simulink model "Test_Bit_Demultiplexer_1_to_4"  (Simulink 8.1)
settings: Solver=ode45  StartTime=0.0  StopTime=len  RelTol=1e-3
libraries: commutil2 x3, Bit_Demultiplexers_Lib x1
settings Model: Creator=N  LastModifiedBy=uzivatel
settings DataIOCC: LimitDataPoints=off  SignalLoggingSaveFormat=Dataset
settings OptimizationCC: ExpressionDepthLimit=128
settings DebuggingCC: UnderspecifiedInitializationDetection=Simplified  MergeDetectMultiDrivingBlocksExec=error  SolverPrmCheckMsg=none  FcnCallInpInsideContextMsg=EnableAllAsError  FrameProcessingCompatibilityMsg=error  StateNameClashWarn=none
settings HardwareCC: ProdBitPerPointer=64  ProdLargestAtomicFloat=Float  ProdIntDivRoundTo=Zero  ProdEndianess=LittleEndian  ProdHWDeviceType=Intel->x86-64 (Windows64)
settings ModelReferenceCC: PropagateSignalLabelsOutOfModel=on
settings GRTTargetCC: CodeReplacementLibrary=None  CombineOutputUpdateFcns=on  CPPClassGenCompliant=on  GRTInterface=off

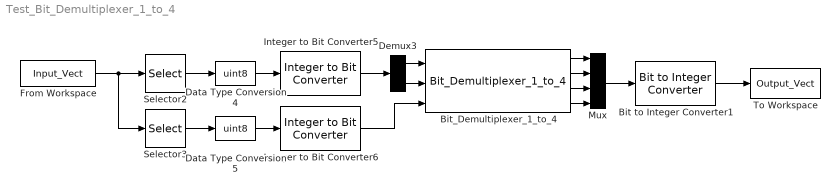
== system Test_Bit_Demultiplexer_1_to_4 ==
  Bit to Integer Converter1 : commutil2/Bit to Integer Converter  nbits=4  bitOrder=MSB first  signedOutputValues=Unsigned  outDtype=uint8  outDtypeSigned=Inherit via internal rule
  Bit_Demultiplexer_1_to_4 : Bit_Demultiplexers_Lib/Bit_Demultiplexers_Lib/Bit_Demultiplexer_1_to_4
  Data Type Conversion4 : DataTypeConversion  OutDataTypeStr=uint8
  Data Type Conversion5 : DataTypeConversion  OutDataTypeStr=uint8
  Demux3 : Demux  Outputs=2
  From Workspace : FromWorkspace  VariableName=Input_Vect  SampleTime=1  Interpolate=off  OutputAfterFinalValue=Holding final value
  Integer to Bit Converter5 : commutil2/Integer to Bit Converter  nbits=2  signedInputValues=Unsigned  bitOrder=MSB first  outDtype=uint8
  Integer to Bit Converter6 : commutil2/Integer to Bit Converter  nbits=1  signedInputValues=Unsigned  bitOrder=MSB first  outDtype=uint8
  Mux : Mux
  Selector2 : Selector  IndexMode=Zero-based  InputPortWidth=2  SampleTime=1  IndexOptions=Index vector (dialog)  Indices=0  OutputSizes=1
  Selector3 : Selector  IndexMode=Zero-based  InputPortWidth=2  IndexOptions=Index vector (dialog)  Indices=1  OutputSizes=1
  To Workspace : ToWorkspace  VariableName=Output_Vect  SampleTime=1
  wires:
  Demux3/1 -> Bit_Demultiplexer_1_to_4/1
  Demux3/2 -> Bit_Demultiplexer_1_to_4/2
  Integer to Bit Converter5/1 -> Demux3/1
  Bit_Demultiplexer_1_to_4/1 -> Mux/1
  Bit_Demultiplexer_1_to_4/2 -> Mux/2
  Bit_Demultiplexer_1_to_4/3 -> Mux/3
  Bit_Demultiplexer_1_to_4/4 -> Mux/4
  Mux/1 -> Bit to Integer Converter1/1
  Bit to Integer Converter1/1 -> To Workspace/1
  From Workspace/1 -> Selector3/1, Selector2/1
  Integer to Bit Converter6/1 -> Bit_Demultiplexer_1_to_4/3
  Selector2/1 -> Data Type Conversion4/1
  Selector3/1 -> Data Type Conversion5/1
  Data Type Conversion4/1 -> Integer to Bit Converter5/1
  Data Type Conversion5/1 -> Integer to Bit Converter6/1
